simulink model "HC_core_demand"  (R2023b)
settings: configuration reference "slow_tsk_conf" (kept outside this file)
undefined symbols (not defined in the file): slow_tsk_st
libraries: eeGeneralControl x2
settings Model: DataDictionary=fmuGenerationDictionay.sldd  ModifiedByFormat=Third Equation Ltd  Creator=Third Equation Ltd  LastModifiedBy=Third Equation Ltd
settings ConfigSetRef: SourceName=slow_tsk_conf

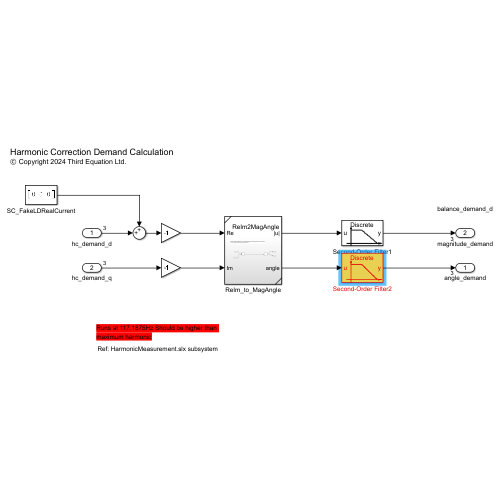
[thumbnail: Simulink's stored preview of the top-level diagram]
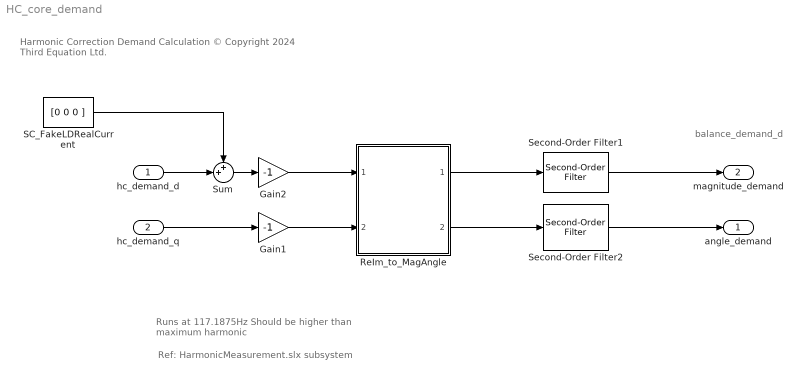
== system HC_core_demand ==
  note: balance_demand_d
  note: Ref: HarmonicMeasurement.slx subsystem
  note: Harmonic Correction Demand Calculation
      | © Copyright 2024 Third Equation Ltd.
  note: Runs at 117.1875Hz Should be higher than
      | maximum harmonic
  hc_demand_d : Inport  OutDataTypeStr=single  PortDimensions=3
  hc_demand_q : Inport  Port=2  OutDataTypeStr=single  PortDimensions=3
  Gain1 : Gain  Gain=-1
  Gain2 : Gain  Gain=-1
  ReIm_to_MagAngle : Subsystem  ReferencedSubsystem=ReIm2MagAngle
  SC_FakeLDRealCurrent : Constant  Value=[0 0 0 ]  OutDataTypeStr=single
  Second-Order Filter1 : eeGeneralControl/Second-Order Filter  FilterType=Low-pass  fn=single(2)  Zeta=single(0.707)  Ts=slow_tsk_st  A0=0  Ph0=0  f0=0  b0=0
  Second-Order Filter2 : eeGeneralControl/Second-Order Filter  FilterType=Low-pass  fn=single(2)  Zeta=single(0.707)  Ts=slow_tsk_st  A0=0  Ph0=0  f0=0  b0=0
  Sum : Sum  Inputs=++|
  angle_demand : Outport  OutDataTypeStr=single  PortDimensions=3
  magnitude_demand : Outport  Port=2  OutDataTypeStr=single  PortDimensions=3
  wires:
  ReIm_to_MagAngle/2 -> Second-Order Filter2/1
  Gain1/1 -> ReIm_to_MagAngle/2
  Second-Order Filter1/1 -> magnitude_demand/1
  Second-Order Filter2/1 -> angle_demand/1
  Gain2/1 -> ReIm_to_MagAngle/1
  hc_demand_q/1 -> Gain1/1
  ReIm_to_MagAngle/1 -> Second-Order Filter1/1
  Sum/1 -> Gain2/1
  SC_FakeLDRealCurrent/1 -> Sum/1
  hc_demand_d/1 -> Sum/2
